simulink model "fuzzy_1"  (R2014b)
settings: Solver=ode45  StartTime=0.0  StopTime=10.0  RelTol=1e-3
libraries: simulink x1, fuzblock x1, powerlib x1
settings Model: Creator=Administrator  LastModifiedBy=Administrator

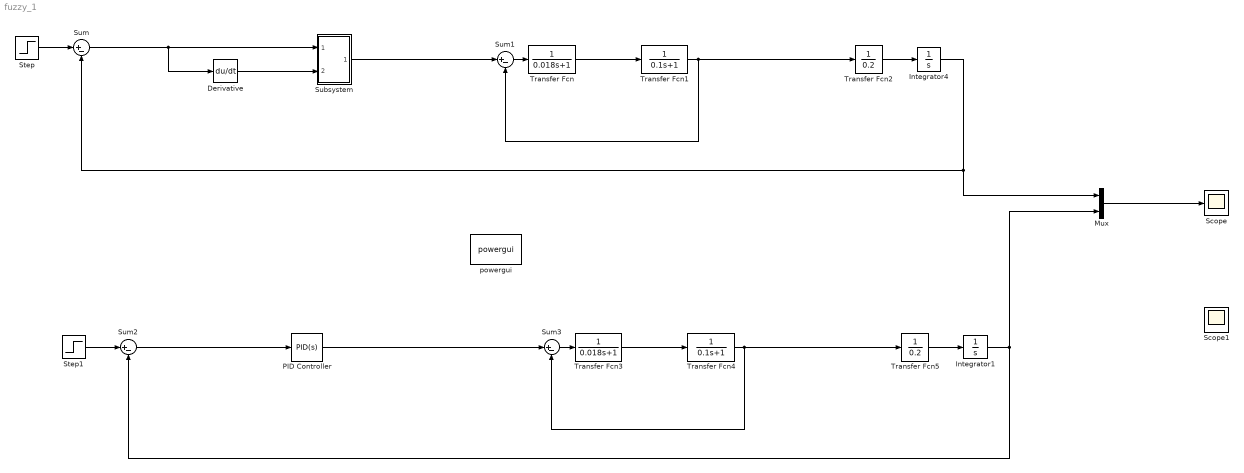
== system fuzzy_1 ==
  Derivative : Derivative
  Integrator1 : Integrator
  Integrator4 : Integrator
  Mux : Mux  Inputs=2
  PID Controller : simulink/Continuous/PID Controller  Controller=PID  TimeDomain=Continuous-time  SampleTime=-1  IntegratorMethod=Forward Euler  FilterMethod=Forward Euler  Form=Parallel  P=12.9851074749726  I=3.96505413373294  D=0.756963167778154  N=4061.73491108422  InitialConditionSource=internal  InitialConditionForIntegrator=0  InitialConditionForFilter=0  ExternalReset=none  LimitOutput=off  UpperSaturationLimit=inf  LowerSaturationLimit=-inf  LinearizeAsGain=on  AntiWindupMode=none  Kb=1  TrackingMode=off  Kt=1  PParamMin=[]  PParamMax=[]  IParamMin=[]  IParamMax=[]  DParamMin=[]  DParamMax=[]  NParamMin=[]  NParamMax=[]  KbParamMin=[]  KbParamMax=[]  KtParamMin=[]  KtParamMax=[]  POutMin=[]  POutMax=[]  IOutMin=[]  IOutMax=[]  DOutMin=[]  DOutMax=[]  NOutMin=[]  NOutMax=[]  KbOutMin=[]  KbOutMax=[]  KtOutMin=[]  KtOutMax=[]  IntegratorOutMin=[]  IntegratorOutMax=[]  FilterOutMin=[]  FilterOutMax=[]  SumOutMin=[]  SumOutMax=[]  SumI1OutMin=[]  SumI1OutMax=[]  SumI2OutMin=[]  SumI2OutMax=[]  SumI3OutMin=[]  SumI3OutMax=[]  SumDOutMin=[]  SumDOutMax=[]  SaturationOutMin=[]  SaturationOutMax=[]  IntegratorContinuousStateAttributes=''  IntegratorStateMustResolveToSignalObject=off  IntegratorRTWStateStorageClass=Auto  FilterContinuousStateAttributes=''  FilterStateMustResolveToSignalObject=off  FilterRTWStateStorageClass=Auto  DifferentiatorICPrevScaledInput=0  DifferentiatorOutMin=[]  DifferentiatorOutMax=[]  UseFilter=on
  Scope : Scope
      settings: YMin=5  YMax=55  SaveName=dianji1
  Scope1 : Scope
      settings: SaveName=dianji
  Step : Step  After=50  SampleTime=0
  Step1 : Step  After=50  SampleTime=0
  Subsystem : Subsystem
  Sum{,1..3} (4 alike) : Sum  Inputs=|+-
  Transfer Fcn : TransferFcn  Denominator=[0.018 1]
  Transfer Fcn1 : TransferFcn  Denominator=[0.1 1]
  Transfer Fcn2 : TransferFcn  Denominator=[0.2]
  Transfer Fcn3 : TransferFcn  Denominator=[0.018 1]
  Transfer Fcn4 : TransferFcn  Denominator=[0.1 1]
  Transfer Fcn5 : TransferFcn  Denominator=[0.2]
  powergui : powerlib/powergui  Priority=1  SimulationMode=Continuous  SolverType=Tustin/Backward Euler (TBE)  SampleTime=50e-6  frequency=60  SPID=off  DisableSnubberDevices=off  DisableRonSwitches=off  DisableVfSwitches=off  SwTol=0  DisplayEquations=off  Interpol=off  methode=off  Ts=100  frequencyindice=60  Pbase=100e6  ErrMax=1e-4  Iterations=50  UnitsV=kV  UnitsW=MW  FunctionMessages=off  echomessages=off  HookPort=off  EnableUseOfTLC=off  x0status=blocks  RestoreLinks=warning  ResistiveCurrentMeasurement=off  Frange=[0:2:500]  Ylog=off  Xlog=on  ShowGrid=off  save=off  variable=ZData  structure=0  ZoomFFT=off  StartTime=0.0  cycles=1  DisplayStyle=1  fundamental=60  FreqAxis=off  MaxFrequency=1000  frequencyindicesteady=1  RmsSteady=1  display=off
  wires:
  Step/1 -> Sum/1
  Transfer Fcn1/1 -> Transfer Fcn2/1, Sum1/2
  Sum1/1 -> Transfer Fcn/1
  Transfer Fcn/1 -> Transfer Fcn1/1
  Transfer Fcn2/1 -> Integrator4/1
  Integrator4/1 -> Mux/1, Sum/2
  Sum/1 -> Derivative/1, Subsystem/1(In1)
  Derivative/1 -> Subsystem/2(In2)
  Step1/1 -> Sum2/1
  Transfer Fcn4/1 -> Transfer Fcn5/1, Sum3/2
  Sum3/1 -> Transfer Fcn3/1
  Transfer Fcn3/1 -> Transfer Fcn4/1
  Transfer Fcn5/1 -> Integrator1/1
  Integrator1/1 -> Sum2/2, Mux/2
  Sum2/1 -> PID Controller/1
  Subsystem/1(Out1) -> Sum1/1
  PID Controller/1 -> Sum3/1
  Mux/1 -> Scope/1

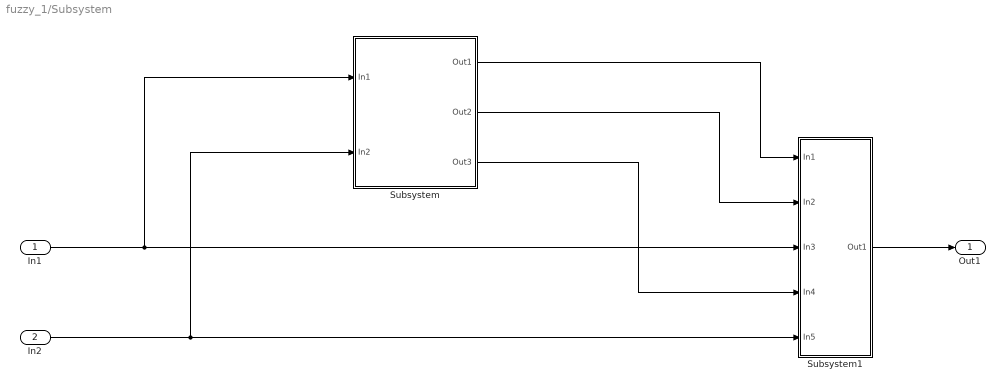
== system fuzzy_1/Subsystem ==
  In1 : Inport
  In2 : Inport  Port=2
  Subsystem : Subsystem
  Subsystem1 : Subsystem
  Out1 : Outport
  wires:
  Subsystem1/1(Out1) -> Out1/1
  In1/1 -> Subsystem/1(In1), Subsystem1/3(In3)
  In2/1 -> Subsystem/2(In2), Subsystem1/5(In5)
  Subsystem/3(Out3) -> Subsystem1/4(In4)
  Subsystem/2(Out2) -> Subsystem1/2(In2)
  Subsystem/1(Out1) -> Subsystem1/1(In1)

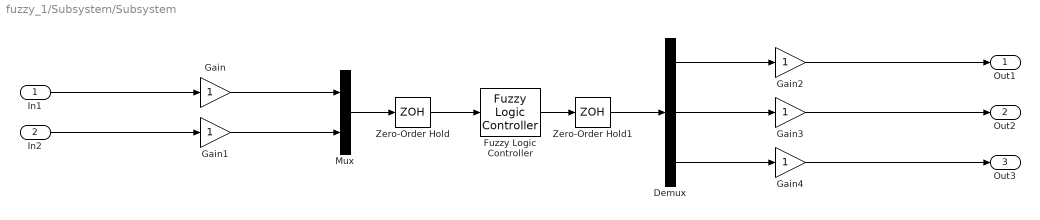
== system fuzzy_1/Subsystem/Subsystem ==
  In1 : Inport
  In2 : Inport  Port=2
  Demux : Demux  Outputs=3
  Fuzzy Logic Controller : fuzblock/Fuzzy Logic  Controller  fis=ceshi
  Gain{,1..4} (5 alike) : Gain
  Mux : Mux  Inputs=2
  Zero-Order Hold : ZeroOrderHold
  Zero-Order Hold1 : ZeroOrderHold
  Out1 : Outport
  Out2 : Outport  Port=2
  Out3 : Outport  Port=3
  wires:
  Mux/1 -> Zero-Order Hold/1
  Fuzzy Logic Controller/1 -> Zero-Order Hold1/1
  Gain1/1 -> Mux/2
  Gain/1 -> Mux/1
  Demux/1 -> Gain2/1
  Demux/2 -> Gain3/1
  Demux/3 -> Gain4/1
  Gain2/1 -> Out1/1
  Gain3/1 -> Out2/1
  Gain4/1 -> Out3/1
  In1/1 -> Gain/1
  In2/1 -> Gain1/1
  Zero-Order Hold/1 -> Fuzzy Logic Controller/1
  Zero-Order Hold1/1 -> Demux/1

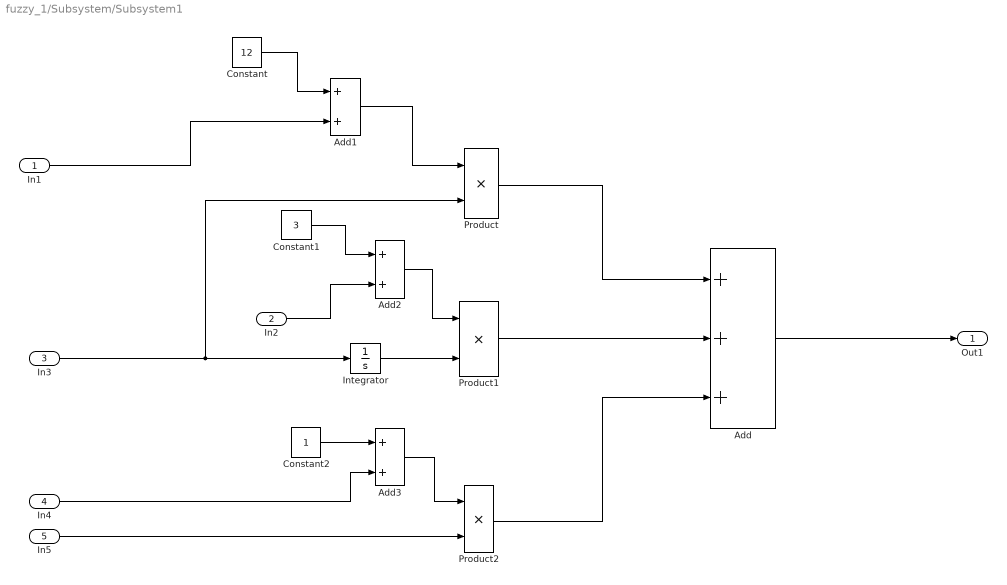
== system fuzzy_1/Subsystem/Subsystem1 ==
  In1 : Inport
  In2 : Inport  Port=2
  In3 : Inport  Port=3
  In4 : Inport  Port=4
  In5 : Inport  Port=5
  Add : Sum  Inputs=+++
  Add1 : Sum
  Add2 : Sum
  Add3 : Sum
  Constant : Constant  Value=12
  Constant1 : Constant  Value=3
  Constant2 : Constant
  Integrator : Integrator
  Product : Product
  Product1 : Product
  Product2 : Product
  Out1 : Outport
  wires:
  Add/1 -> Out1/1
  Product/1 -> Add/1
  Product1/1 -> Add/2
  Product2/1 -> Add/3
  In3/1 -> Product/2, Integrator/1
  Integrator/1 -> Product1/2
  In5/1 -> Product2/2
  Constant/1 -> Add1/1
  Constant1/1 -> Add2/1
  Constant2/1 -> Add3/1
  Add1/1 -> Product/1
  Add2/1 -> Product1/1
  Add3/1 -> Product2/1
  In1/1 -> Add1/2
  In2/1 -> Add2/2
  In4/1 -> Add3/2
